simulink model "CryoDet12Chan"  (R2016b)
settings: Solver=ode45  StartTime=0.0  StopTime=10e-4  MaxStep=1e-9  RelTol=1e-3
values from neighbouring files (symbols this model uses):
  Fclk = Fadc/2    (= 153600000)    [setupCryoFPGA.m]    (also in setupCryoNew.m)
  freqBusAddrBits = 4    [setupCryoFPGA.m]    (also in setupCryoNew.m)
  noise = exp(2i*pi*rand(1, noiseLen))    [setupCryoFPGA.m]    (also in setupCryoNew.m)
  noiseLen = 128    [setupCryoFPGA.m]    (also in setupCryoNew.m)
  noiseSteps = 32    [setupCryoFPGA.m]    (also in setupCryoNew.m)
  notch = tf( [1 a*wNotch/Q wNotch^2], [1 wNotch/Q wNotch^2])    [setupCryoFPGA.m]    (also in setupCryoNew.m)
  notch2 = tf( [1 a*wNotch/Q wNotch^2], [1 wNotch/Q wNotch^2])    [setupCryoFPGA.m]    (also in setupCryoNew.m)
  notch3 = tf( [1 a*wNotch/Q wNotch^2], [1 wNotch/Q wNotch^2])    [setupCryoFPGA.m]    (also in setupCryoNew.m)
  notch4 = tf( [1 a*wNotch/Q wNotch^2], [1 wNotch/Q wNotch^2])    [setupCryoFPGA.m]    (also in setupCryoNew.m)
  Tclk = 1/Fclk    (= 6.51041666667e-09)    [setupCryoFPGA.m]    (also in setupCryoNew.m)
undefined symbols (not defined in the file or in its folder): AXI4, Lite, xlipgetpartsetting
libraries: xbsIndex_r4 x1191
(part 3 of 9)

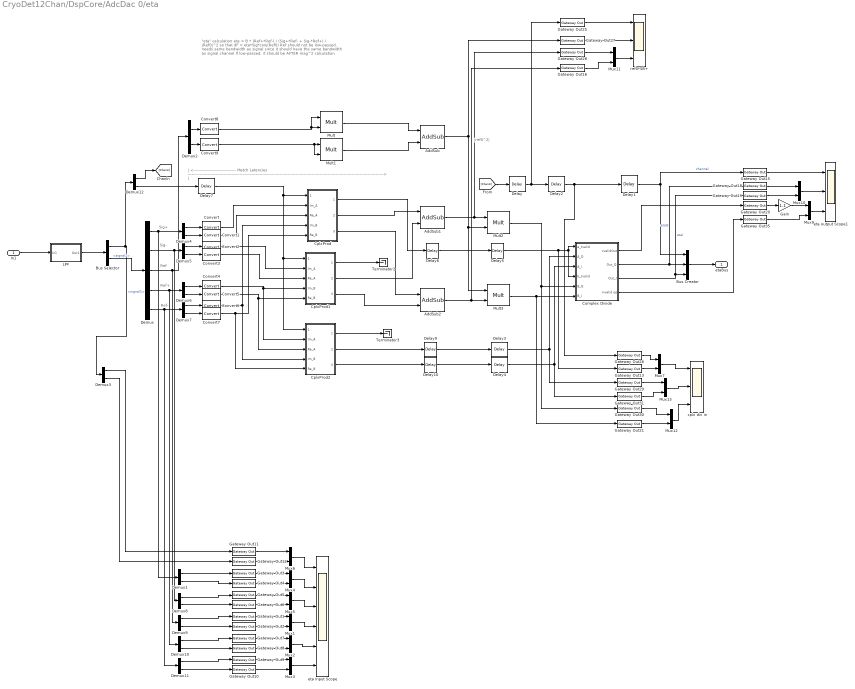
== system CryoDet12Chan/DspCore/AdcDac 0/eta ==
  note: Sig+
  note: Sig-
  note: Ref+
  note: "eta" calculation
      |
      | eta = B * (Ref+*Ref-) / (Sig+*Ref- + Sig-*Ref+) / |Ref0|^2
      |
      | so that dF = eta*Sig*conj(Ref0)
      |
      | Ref should not be low-passed, needs same bandwidth as signal since it should have the same bandwidth as signal channel
      | If low-passed, it should be AFTER mag^2 calculation
  note: Ref
  note: Ref-
  note: | <-------------------------------- Match Latencies ---------------------------------------------------------------------------------------------------------------------------------------------------> |
  note: |ref0^2|
  In1 : Inport
  AddSub : xbsIndex_r4/AddSub  mode=Addition  use_carryin=off  use_carryout=off  en=off  latency=3  precision=Full  arith_type=Unsigned  n_bits=32  bin_pt=30  quantization="Round  (unbiased: +/- Inf)"  overflow=Saturate  use_behavioral_HDL=off  hw_selection=DSP48  pipelined=on  dbl_ovrd=off  block_type=addsub
  AddSub1 : xbsIndex_r4/AddSub  mode=Addition  use_carryin=off  use_carryout=off  en=off  latency=3  precision=Full  arith_type="Signed  (2's comp)"  n_bits=32  bin_pt=30  quantization="Round  (unbiased: +/- Inf)"  overflow=Saturate  use_behavioral_HDL=off  hw_selection=DSP48  pipelined=on  dbl_ovrd=off  block_type=addsub
  AddSub2 : xbsIndex_r4/AddSub  mode=Addition  use_carryin=off  use_carryout=off  en=off  latency=3  precision=Full  arith_type="Signed  (2's comp)"  n_bits=32  bin_pt=30  quantization="Round  (unbiased: +/- Inf)"  overflow=Saturate  use_behavioral_HDL=off  hw_selection=DSP48  pipelined=on  dbl_ovrd=off  block_type=addsub
  Bus Creator : BusCreator  Inputs=3
  Bus Selector : BusSelector  OutputSignals=signal1,signal2
  Complex Divide : Subsystem
  Convert{,1..9} (10 alike) : xbsIndex_r4/Convert  gui_display_data_type=Floating-point  arith_type=Floating-point  n_bits=16  bin_pt=14  float_type=Single  exp_bits=8  fraction_bits=24  quantization=Truncate  overflow=Wrap  en=off  latency=1  pipeline=off  dbl_ovrd=off  block_type=convert
  CplxProd : Subsystem
  CplxProd1 : Subsystem
  CplxProd2 : Subsystem
  Delay : xbsIndex_r4/Delay  rst=off  infoeditControl=Selection of Reset will increase slice count due to use of real FFs and instead of SRLs  en=off  latency=10  reg_retiming=off  dbl_ovrd=off  block_type=delay
  Delay1 : xbsIndex_r4/Delay  rst=off  infoeditControl=Selection of Reset will increase slice count due to use of real FFs and instead of SRLs  en=off  latency=17  reg_retiming=on  dbl_ovrd=off  block_type=delay
  Delay{2..6,9..10} (7 alike) : xbsIndex_r4/Delay  rst=off  infoeditControl=Selection of Reset will increase slice count due to use of real FFs and instead of SRLs  en=off  latency=3  reg_retiming=off  dbl_ovrd=off  block_type=delay
  Delay7 : xbsIndex_r4/Delay  rst=off  infoeditControl=Selection of Reset will increase slice count due to use of real FFs and instead of SRLs  en=off  latency=1  reg_retiming=off  dbl_ovrd=off  block_type=delay
  Demux : Demux  Outputs=5
  Demux{1..12} (12 alike) : Demux  Outputs=2
  Gain : Gain  Gain=1.1
  Gateway Out{1..13,15..16,18..21,25..31,35} (27 alike) : xbsIndex_r4/Gateway Out  inherit_from_input=off  hdl_port=off  rows=1  columns=1  UseAsDAC=off  DACChannel='1'  interface=None  automatic_assignment=on  address_offset=hex2dec('00')  intf_name=''  intf_description=''  timing_constraint=None  locs_specified=off  LOCs={}  io_standard={}  block_type=gatewayout
  LPF : Subsystem
  Mult : xbsIndex_r4/Mult  precision=Full  arith_type="Signed  (2's comp)"  n_bits=32  bin_pt=30  quantization="Round  (unbiased: +/- Inf)"  overflow=Saturate  en=off  latency=6  use_behavioral_HDL=off  opt=Speed  use_embedded=on  optimum_pipeline=off  pipeline=on  dbl_ovrd=off  use_rpm=on  placement_style=Triangular  block_type=mult
  Mult1 : xbsIndex_r4/Mult  precision=Full  arith_type="Signed  (2's comp)"  n_bits=32  bin_pt=30  quantization="Round  (unbiased: +/- Inf)"  overflow=Saturate  en=off  latency=6  use_behavioral_HDL=off  opt=Speed  use_embedded=on  optimum_pipeline=off  pipeline=on  dbl_ovrd=off  use_rpm=on  placement_style=Triangular  block_type=mult
  Mult2 : xbsIndex_r4/Mult  precision=Full  arith_type="Signed  (2's comp)"  n_bits=32  bin_pt=30  quantization="Round  (unbiased: +/- Inf)"  overflow=Saturate  en=off  latency=3  use_behavioral_HDL=off  opt=Speed  use_embedded=on  optimum_pipeline=off  pipeline=on  dbl_ovrd=off  use_rpm=on  placement_style=Triangular  block_type=mult
  Mult3 : xbsIndex_r4/Mult  precision=Full  arith_type="Signed  (2's comp)"  n_bits=32  bin_pt=30  quantization="Round  (unbiased: +/- Inf)"  overflow=Saturate  en=off  latency=3  use_behavioral_HDL=off  opt=Speed  use_embedded=on  optimum_pipeline=off  pipeline=on  dbl_ovrd=off  use_rpm=on  placement_style=Triangular  block_type=mult
  Mux{1..7,9..13} (12 alike) : Mux  Inputs=2
  Terminator2 : Terminator
  Terminator3 : Terminator
  cplx div in : Scope  NumInputPorts=3
  eta Input Scope : Scope  NumInputPorts=6
  eta output Scope1 : Scope  NumInputPorts=3
  ref0*SB+ : Scope  NumInputPorts=3
  etaBus : Outport
  wires:
  Demux4/1 -> Convert/1
  Demux4/2 -> Convert1/1
  Demux7/1 -> Convert6/1
  Demux7/2 -> Convert7/1
  Demux5/1 -> Convert2/1
  Demux5/2 -> Convert3/1
  Demux6/1 -> Convert4/1
  Demux6/2 -> Convert5/1
  Demux12/2 -> Delay7/1
  AddSub2/1 -> Gateway Out16/1, Mult3/2
  AddSub1/1 -> Gateway Out28/1, Mult2/1
  Mult/1 -> AddSub/1
  Mult1/1 -> AddSub/2
  Demux2/1 -> Convert8/1
  Demux2/2 -> Convert9/1
  CplxProd1/3(Re_Out) -> AddSub2/2
  CplxProd/3(Re_Out) -> AddSub2/1
  CplxProd1/2(Im_Out) -> AddSub1/2
  AddSub/1 -> Mult3/1, Mult2/2, Gateway Out27/1
  Mult2/1 -> Complex Divide/5(B_Q), Gateway Out30/1
  Mult3/1 -> Gateway Out21/1, Complex Divide/6(B_I)
  CplxProd/1(tvalidOut) -> Delay6/1
  CplxProd2/3(Re_Out) -> Delay10/1
  In1/1 -> LPF/1(In1)
  Bus Selector/2 -> Demux/1  "<signal2>"
  [ChanIn] -> Delay/1
  Delay/1 -> Gateway Out25/1, Delay2/1
  LPF/1(Out1) -> Bus Selector/1
  Delay1/1 -> Gateway Out15/1, Bus Creator/1  "channel"
  Complex Divide/2(Out_Q) -> Gateway Out18/1, Bus Creator/2  "etaQ"
  Complex Divide/3(Out_I) -> Gateway Out19/1, Bus Creator/3  "etaI"
  Bus Creator/1 -> etaBus/1
  Bus Selector/1 -> Demux12/1, Demux3/1  "<signal1>"
  Demux3/1 -> Gateway Out11/1
  Demux3/2 -> Gateway Out12/1
  Demux/5 -> Demux11/1, Demux7/1
  Demux/4 -> Demux6/1, Demux10/1
  Demux/2 -> Demux8/1, Demux5/1
  Demux/1 -> Demux4/1, Demux1/1
  Demux/3 -> Demux9/1, Demux2/1
  CplxProd1/1(tvalidOut) -> Terminator2/1
  Gateway Out6/1 -> Mux5/2
  Gateway Out5/1 -> Mux5/1
  Gateway Out4/1 -> Mux4/2
  Gateway Out3/1 -> Mux4/1
  Mux4/1 -> eta Input Scope/2
  Mux5/1 -> eta Input Scope/3
  Gateway Out2/1 -> Mux1/2
  Gateway Out1/1 -> Mux1/1
  Gateway Out8/1 -> Mux2/2
  Gateway Out7/1 -> Mux2/1
  Gateway Out10/1 -> Mux3/2
  Gateway Out9/1 -> Mux3/1
  Mux3/1 -> eta Input Scope/6
  Mux2/1 -> eta Input Scope/5
  Mux1/1 -> eta Input Scope/4
  Demux1/1 -> Gateway Out3/1
  Demux1/2 -> Gateway Out4/1
  Demux8/2 -> Gateway Out6/1
  Demux8/1 -> Gateway Out5/1
  Demux9/2 -> Gateway Out2/1
  Demux9/1 -> Gateway Out1/1
  Demux10/2 -> Gateway Out8/1
  Demux10/1 -> Gateway Out7/1
  Demux11/2 -> Gateway Out10/1
  Demux11/1 -> Gateway Out9/1
  Gateway Out12/1 -> Mux6/2
  Gateway Out11/1 -> Mux6/1
  Mux6/1 -> eta Input Scope/1
  Gateway Out19/1 -> Mux10/2
  Gateway Out18/1 -> Mux10/1
  Mux10/1 -> eta output Scope1/2
  Gateway Out15/1 -> eta output Scope1/1
  Gateway Out25/1 -> ref0*SB+/1
  Gateway Out27/1 -> ref0*SB+/2
  Mux11/1 -> ref0*SB+/3
  Gateway Out28/1 -> Mux11/1
  Gateway Out16/1 -> Mux11/2
  Delay2/1 -> Gateway Out26/1, Delay1/1
  Delay3/1 -> Complex Divide/2(A_Q), Gateway Out29/1
  Delay4/1 -> Complex Divide/3(A_I), Gateway Out31/1
  Mux12/1 -> cplx div in/3
  Gateway Out30/1 -> Mux12/1
  Gateway Out21/1 -> Mux12/2
  Gateway Out29/1 -> Mux13/1
  Mux13/1 -> cplx div in/2
  Gateway Out31/1 -> Mux13/2
  Gateway Out13/1 -> Mux7/2
  Gateway Out26/1 -> Mux7/1
  Mux7/1 -> cplx div in/1
  Demux12/1 -> [ChanIn]
  CplxProd/2(Im_Out) -> AddSub1/1
  Gateway Out20/1 -> Gain/1
  Gateway Out35/1 -> Mux9/2
  Complex Divide/4(invalid op) -> Gateway Out35/1
  Mux9/1 -> eta output Scope1/3
  Gain/1 -> Mux9/1
  Convert/1 -> CplxProd/2(Im_A)
  Convert1/1 -> CplxProd/3(Re_A)
  Convert2/1 -> CplxProd1/2(Im_A)
  Convert3/1 -> CplxProd1/3(Re_A)
  Convert4/1 -> CplxProd2/2(Im_A), CplxProd1/4(Im_B)
  Convert5/1 -> CplxProd2/3(Re_A), CplxProd1/5(Re_B)
  Convert6/1 -> CplxProd2/4(Im_B), CplxProd/4(Im_B)
  Convert7/1 -> CplxProd2/5(Re_B), CplxProd/5(Re_B)
  Convert9/1 -> Mult1/2, Mult1/1
  Convert8/1 -> Mult/1, Mult/2
  Delay6/1 -> Delay5/1
  Delay7/1 -> CplxProd/1(tvalidIn), CplxProd1/1(tvalidIn), CplxProd2/1(tvalidIn)
  CplxProd2/1(tvalidOut) -> Terminator3/1
  Delay10/1 -> Delay4/1
  Delay9/1 -> Delay3/1
  CplxProd2/2(Im_Out) -> Delay9/1
  Delay5/1 -> Gateway Out13/1, Complex Divide/4(b_tvalid), Complex Divide/1(a_tvalid)
  Complex Divide/1(tvalidOut) -> Gateway Out20/1

== system CryoDet12Chan/DspCore/AdcDac 0/loopFilter ==
  note: convert to MHz
  note: F out should be Fi + DF
      | where DF is integral of frequency error dF subject to limits and FBen
  note: loopFilter
      | multi-line feedback block
      | mplement intial frequency, limits, integrator, gain
  In1 : Inport
  Assert : xbsIndex_r4/Assert  assert_type=on  type_source=Explicitly  gui_display_data_type=Fixed-point  arith_type=Unsigned  n_bits=4  bin_pt=0  preci_type=Single  exp_width=8  frac_width=24  assert_rate=on  rate_source=Explicitly  period=Tclk  output_port=on  block_type=assert
  Assert1 : xbsIndex_r4/Assert  assert_type=on  type_source=Explicitly  gui_display_data_type=Fixed-point  arith_type="Signed  (2's comp)"  n_bits=32  bin_pt=30  preci_type=Single  exp_width=8  frac_width=24  assert_rate=on  rate_source=Explicitly  period=Tclk  output_port=on  block_type=assert
  Assert2 : xbsIndex_r4/Assert  assert_type=on  type_source=Explicitly  gui_display_data_type=Boolean  arith_type=Boolean  n_bits=16  bin_pt=14  preci_type=Single  exp_width=8  frac_width=24  assert_rate=on  rate_source=Explicitly  period=Tclk  output_port=on  block_type=assert
  Assert5 : xbsIndex_r4/Assert  assert_type=on  type_source=Explicitly  gui_display_data_type=Fixed-point  arith_type=Unsigned  n_bits=25  bin_pt=0  preci_type=Single  exp_width=8  frac_width=24  assert_rate=on  rate_source=Explicitly  period=Tclk  output_port=on  block_type=assert
  Assert6 : xbsIndex_r4/Assert  assert_type=on  type_source=Explicitly  gui_display_data_type=Fixed-point  arith_type=Unsigned  n_bits=16  bin_pt=16  preci_type=Single  exp_width=8  frac_width=24  assert_rate=on  rate_source=Explicitly  period=Tclk  output_port=on  block_type=assert
  Assert8 : xbsIndex_r4/Assert  assert_type=on  type_source=Explicitly  gui_display_data_type=Fixed-point  arith_type=Unsigned  n_bits=24  bin_pt=24  preci_type=Single  exp_width=8  frac_width=24  assert_rate=on  rate_source=Explicitly  period=Tclk  output_port=on  block_type=assert
  Assert9 : xbsIndex_r4/Assert  assert_type=on  type_source=Explicitly  gui_display_data_type=Fixed-point  arith_type=Unsigned  n_bits=4  bin_pt=0  preci_type=Single  exp_width=8  frac_width=24  assert_rate=on  rate_source=Explicitly  period=Tclk  output_port=on  block_type=assert
  Bus Selector : BusSelector  OutputSignals=channel,freqError
  Concat : xbsIndex_r4/Concat  num_inputs=2  dbl_ovrd=off  block_type=concat
  Constant : xbsIndex_r4/Constant  const=0  gui_display_data_type=Fixed-point  arith_type=Unsigned  n_bits=4  bin_pt=0  preci_type=Single  exp_width=8  frac_width=24  explicit_period=off  period=1  equ=P=C  opselect=C  inp2=PCIN>>17  opr=+  inp1=P  carry=CIN  dbl_ovrd=off  block_type=constant
  Constant1 : xbsIndex_r4/Constant  const=0  gui_display_data_type=Fixed-point  arith_type=Unsigned  n_bits=4  bin_pt=0  preci_type=Single  exp_width=8  frac_width=24  explicit_period=off  period=1  equ=P=C  opselect=C  inp2=PCIN>>17  opr=+  inp1=P  carry=CIN  dbl_ovrd=off  block_type=constant
  Constant2 : xbsIndex_r4/Constant  const=1  gui_display_data_type=Fixed-point  arith_type=Unsigned  n_bits=4  bin_pt=0  preci_type=Single  exp_width=8  frac_width=24  explicit_period=off  period=1  equ=P=C  opselect=C  inp2=PCIN>>17  opr=+  inp1=P  carry=CIN  dbl_ovrd=off  block_type=constant
  Delay2 : xbsIndex_r4/Delay  rst=off  infoeditControl=Selection of Reset will increase slice count due to use of real FFs and instead of SRLs  en=off  latency=3  reg_retiming=off  dbl_ovrd=off  block_type=delay
  Delay3 : xbsIndex_r4/Delay  rst=off  infoeditControl=Selection of Reset will increase slice count due to use of real FFs and instead of SRLs  en=off  latency=3  reg_retiming=off  dbl_ovrd=off  block_type=delay
  Display2 : Display
  Display3 : Display
  Gain1 : Gain  Gain=185
  Gain2 : Gain  Gain=185
  Gain3 : Gain  Gain=185
  Gateway Out12 : xbsIndex_r4/Gateway Out  inherit_from_input=off  hdl_port=off  rows=1  columns=1  UseAsDAC=off  DACChannel='1'  interface=None  automatic_assignment=on  address_offset=hex2dec('00')  intf_name=''  intf_description=''  timing_constraint=None  locs_specified=off  LOCs={}  io_standard={}  block_type=gatewayout
  Gateway Out13 : xbsIndex_r4/Gateway Out  inherit_from_input=on  hdl_port=off  rows=1  columns=1  UseAsDAC=off  DACChannel='1'  interface=None  automatic_assignment=on  address_offset=hex2dec('00')  intf_name=''  intf_description=''  timing_constraint=None  locs_specified=off  LOCs={}  io_standard={}  block_type=gatewayout
  Gateway Out3 : xbsIndex_r4/Gateway Out  inherit_from_input=off  hdl_port=off  rows=1  columns=1  UseAsDAC=off  DACChannel='1'  interface=None  automatic_assignment=on  address_offset=hex2dec('00')  intf_name=''  intf_description=''  timing_constraint=None  locs_specified=off  LOCs={}  io_standard={}  block_type=gatewayout
  Gateway Out4 : xbsIndex_r4/Gateway Out  inherit_from_input=off  hdl_port=off  rows=1  columns=1  UseAsDAC=off  DACChannel='1'  interface=None  automatic_assignment=on  address_offset=hex2dec('00')  intf_name=''  intf_description=''  timing_constraint=None  locs_specified=off  LOCs={}  io_standard={}  block_type=gatewayout
  Gateway Out5 : xbsIndex_r4/Gateway Out  inherit_from_input=on  hdl_port=off  rows=1  columns=1  UseAsDAC=off  DACChannel='1'  interface=None  automatic_assignment=on  address_offset=hex2dec('00')  intf_name=''  intf_description=''  timing_constraint=None  locs_specified=off  LOCs={}  io_standard={}  block_type=gatewayout
  Logical : xbsIndex_r4/Logical  logical_function=OR  inputs=2  en=off  latency=3  precision=User Defined  arith_type=Boolean  n_bits=16  bin_pt=0  align_bp=on  dbl_ovrd=off  block_type=logical
  MCode : xbsIndex_r4/MCode  mfname=multiLineFeedbackpipelined  explicit_period=on  period=Tclk  inputsTable={'boundInpExpr'=>['','','','',''],'inputs'=>['channelNo','deltaF','FBen','Finitial','dFmax']}  outputsTable={'outputs'=>['freq','chanOut'],'suppressOut'=>['off','off']}  enable_stdout=off  enable_debug=off  suppress_output=on  defparams={}  hide_port_list={}  dbl_ovrd=off  block_type=mcode
  Mult : xbsIndex_r4/Mult  precision=User Defined  arith_type="Signed  (2's comp)"  n_bits=32  bin_pt=30  quantization=Truncate  overflow=Saturate  en=off  latency=3  use_behavioral_HDL=off  opt=Speed  use_embedded=on  optimum_pipeline=off  pipeline=on  dbl_ovrd=off  use_rpm=on  placement_style=Triangular  block_type=mult
  Mux : xbsIndex_r4/Mux  inputs=2  en=off  latency=1  precision=Full  arith_type=Unsigned  n_bits=16  bin_pt=14  quantization=Truncate  overflow=Wrap  dbl_ovrd=off  block_type=mux
  Negate : xbsIndex_r4/Negate  precision=Full  arith_type=Unsigned  n_bits=16  bin_pt=14  quantization=Truncate  overflow=Wrap  en=off  latency=1  dbl_ovrd=off  block_type=negate
  Register : xbsIndex_r4/Register  init=0  rst=off  en=on  dbl_ovrd=off  block_type=register
  Register1 : xbsIndex_r4/Register  init=0  rst=off  en=on  dbl_ovrd=off  block_type=register
  Register2 : xbsIndex_r4/Register  init=0  rst=off  en=on  dbl_ovrd=off  block_type=register
  Reinterpret : xbsIndex_r4/Reinterpret  force_arith_type=off  arith_type=Unsigned  force_bin_pt=on  bin_pt=0  block_type=reinterpret
  Relational : xbsIndex_r4/Relational  mode=a=b  op_type=Bool  en=off  latency=0  dbl_ovrd=off  block_type=relational
  Relational1 : xbsIndex_r4/Relational  mode=a=b  op_type=Bool  en=off  latency=0  dbl_ovrd=off  block_type=relational
  Relational2 : xbsIndex_r4/Relational  mode=a=b  op_type=Bool  en=off  latency=0  dbl_ovrd=off  block_type=relational
  initial Frequencies : Subsystem
  loop filter input : Scope  NumInputPorts=2
  loop filter output : Scope  NumInputPorts=3
  Out1 : Outport
  tag scope: freqBus=global
  wires:
  In1/1 -> Bus Selector/1
  Bus Selector/1 -> Relational/1, Gateway Out3/1, initial Frequencies/1(channel), Delay3/1  "<channel>"
  Bus Selector/2 -> Mult/1, Register/1  "<freqError>"
  MCode/2 -> Assert9/1, Relational2/2, Gateway Out12/1, Relational1/2  "channel"
  MCode/1 -> Assert8/1, Register2/1, Register1/1  "frequency"
  Concat/1 -> [freqBus], Out1/1
  [fbPolarity] -> Mux/1
  [FBgain] -> Mux/2, Negate/1
  [FBlimit] -> Assert6/1
  initial Frequencies/1(Fi) -> Delay2/1
  Assert/1 -> MCode/1
  Assert1/1 -> MCode/2
  Assert2/1 -> MCode/3
  Assert5/1 -> MCode/4
  Assert6/1 -> MCode/5
  Assert9/1 -> Concat/1
  Assert8/1 -> Reinterpret/1
  Reinterpret/1 -> Concat/2
  Gateway Out13/1 -> Gain1/1
  Gateway Out12/1 -> loop filter output/1
  Gateway Out4/1 -> Gain2/1
  Gateway Out3/1 -> loop filter input/1, Display2/1
  Constant/1 -> Relational/2
  Relational/1 -> Register/2
  Register/1 -> Gateway Out4/1
  Constant1/1 -> Relational1/1
  Relational1/1 -> Register1/2
  Register1/1 -> Gateway Out13/1
  Gain1/1 -> loop filter output/2
  Gain2/1 -> Display3/1, loop filter input/2
  Constant2/1 -> Relational2/1
  Relational2/1 -> Register2/2
  Register2/1 -> Gateway Out5/1
  Gateway Out5/1 -> Gain3/1
  Gain3/1 -> loop filter output/3
  Negate/1 -> Mux/3
  Mult/1 -> Assert1/1
  Mux/1 -> Mult/2
  [fpgaReset] -> Logical/2
  [FBen] -> Logical/1
  Logical/1 -> Assert2/1
  Delay3/1 -> Assert/1
  Delay2/1 -> Assert5/1

== system CryoDet12Chan/DspCore/AdcDac 0/twelveLineUDC 0 ==
  In1 : Inport
  BDC scope : Scope  NumInputPorts=2
  Constant : xbsIndex_r4/Constant  const=0  gui_display_data_type=Fixed-point  arith_type=Unsigned  n_bits=4  bin_pt=0  preci_type=Single  exp_width=8  frac_width=24  explicit_period=off  period=1  equ=P=C  opselect=C  inp2=PCIN>>17  opr=+  inp1=P  carry=CIN  dbl_ovrd=off  block_type=constant
  Constant1 : xbsIndex_r4/Constant  const=1  gui_display_data_type=Fixed-point  arith_type=Unsigned  n_bits=4  bin_pt=0  preci_type=Single  exp_width=8  frac_width=24  explicit_period=off  period=1  equ=P=C  opselect=C  inp2=PCIN>>17  opr=+  inp1=P  carry=CIN  dbl_ovrd=off  block_type=constant
  Constant10 : xbsIndex_r4/Constant  const=10  gui_display_data_type=Fixed-point  arith_type=Unsigned  n_bits=4  bin_pt=0  preci_type=Single  exp_width=8  frac_width=24  explicit_period=off  period=1  equ=P=C  opselect=C  inp2=PCIN>>17  opr=+  inp1=P  carry=CIN  dbl_ovrd=off  block_type=constant
  Constant11 : xbsIndex_r4/Constant  const=11  gui_display_data_type=Fixed-point  arith_type=Unsigned  n_bits=4  bin_pt=0  preci_type=Single  exp_width=8  frac_width=24  explicit_period=off  period=1  equ=P=C  opselect=C  inp2=PCIN>>17  opr=+  inp1=P  carry=CIN  dbl_ovrd=off  block_type=constant
  Constant12 : xbsIndex_r4/Constant  const=15  gui_display_data_type=Fixed-point  arith_type=Unsigned  n_bits=4  bin_pt=0  preci_type=Single  exp_width=8  frac_width=24  explicit_period=off  period=1  equ=P=C  opselect=C  inp2=PCIN>>17  opr=+  inp1=P  carry=CIN  dbl_ovrd=off  block_type=constant
  Constant2 : xbsIndex_r4/Constant  const=2  gui_display_data_type=Fixed-point  arith_type=Unsigned  n_bits=4  bin_pt=0  preci_type=Single  exp_width=8  frac_width=24  explicit_period=off  period=1  equ=P=C  opselect=C  inp2=PCIN>>17  opr=+  inp1=P  carry=CIN  dbl_ovrd=off  block_type=constant
  Constant3 : xbsIndex_r4/Constant  const=3  gui_display_data_type=Fixed-point  arith_type=Unsigned  n_bits=4  bin_pt=0  preci_type=Single  exp_width=8  frac_width=24  explicit_period=off  period=1  equ=P=C  opselect=C  inp2=PCIN>>17  opr=+  inp1=P  carry=CIN  dbl_ovrd=off  block_type=constant
  Constant4 : xbsIndex_r4/Constant  const=4  gui_display_data_type=Fixed-point  arith_type=Unsigned  n_bits=4  bin_pt=0  preci_type=Single  exp_width=8  frac_width=24  explicit_period=off  period=1  equ=P=C  opselect=C  inp2=PCIN>>17  opr=+  inp1=P  carry=CIN  dbl_ovrd=off  block_type=constant
  Constant5 : xbsIndex_r4/Constant  const=5  gui_display_data_type=Fixed-point  arith_type=Unsigned  n_bits=4  bin_pt=0  preci_type=Single  exp_width=8  frac_width=24  explicit_period=off  period=1  equ=P=C  opselect=C  inp2=PCIN>>17  opr=+  inp1=P  carry=CIN  dbl_ovrd=off  block_type=constant
  Constant6 : xbsIndex_r4/Constant  const=6  gui_display_data_type=Fixed-point  arith_type=Unsigned  n_bits=4  bin_pt=0  preci_type=Single  exp_width=8  frac_width=24  explicit_period=off  period=1  equ=P=C  opselect=C  inp2=PCIN>>17  opr=+  inp1=P  carry=CIN  dbl_ovrd=off  block_type=constant
  Constant7 : xbsIndex_r4/Constant  const=7  gui_display_data_type=Fixed-point  arith_type=Unsigned  n_bits=4  bin_pt=0  preci_type=Single  exp_width=8  frac_width=24  explicit_period=off  period=1  equ=P=C  opselect=C  inp2=PCIN>>17  opr=+  inp1=P  carry=CIN  dbl_ovrd=off  block_type=constant
  Constant8 : xbsIndex_r4/Constant  const=8  gui_display_data_type=Fixed-point  arith_type=Unsigned  n_bits=4  bin_pt=0  preci_type=Single  exp_width=8  frac_width=24  explicit_period=off  period=1  equ=P=C  opselect=C  inp2=PCIN>>17  opr=+  inp1=P  carry=CIN  dbl_ovrd=off  block_type=constant
  Constant9 : xbsIndex_r4/Constant  const=9  gui_display_data_type=Fixed-point  arith_type=Unsigned  n_bits=4  bin_pt=0  preci_type=Single  exp_width=8  frac_width=24  explicit_period=off  period=1  equ=P=C  opselect=C  inp2=PCIN>>17  opr=+  inp1=P  carry=CIN  dbl_ovrd=off  block_type=constant
  Counter : xbsIndex_r4/Counter  cnt_type=Count Limited  cnt_to=15  operation=Up  start_count=0  cnt_by_val=1  arith_type=Unsigned  n_bits=4  bin_pt=0  load_pin=off  rst=on  en=on  explicit_period=off  period=Tclk  use_behavioral_HDL=off  implementation=Fabric  dbl_ovrd=off  block_type=counter
  DAC Sum : Subsystem
  Delay : xbsIndex_r4/Delay  rst=off  infoeditControl=Selection of Reset will increase slice count due to use of real FFs and instead of SRLs  en=off  latency=6  reg_retiming=off  dbl_ovrd=off  block_type=delay
  Demux : Demux
  Gateway Out{1,7..10,23} (6 alike) : xbsIndex_r4/Gateway Out  inherit_from_input=off  hdl_port=off  rows=1  columns=1  UseAsDAC=off  DACChannel='1'  interface=None  automatic_assignment=on  address_offset=hex2dec('00')  intf_name=''  intf_description=''  timing_constraint=None  locs_specified=off  LOCs={}  io_standard={}  block_type=gatewayout
  Mux12X4 : Subsystem
  Mux6 : Mux  Inputs=2
  Mux7 : Mux  Inputs=2
  Relational : xbsIndex_r4/Relational  mode=a!=b  op_type=Bool  en=off  latency=0  dbl_ovrd=off  block_type=relational
  SBdemod : Subsystem
  Toolbar : xbsIndex_r4/Toolbar  func=xltoolbar  block_type=toolbar
      settings: infoedit=Toolbar
  oneLineUpDown0 : Subsystem
  oneLineUpDown1 : Subsystem
  oneLineUpDown10 : Subsystem
  oneLineUpDown11 : Subsystem
  oneLineUpDown2 : Subsystem
  oneLineUpDown3 : Subsystem
  oneLineUpDown4 : Subsystem
  oneLineUpDown5 : Subsystem
  oneLineUpDown6 : Subsystem
  oneLineUpDown7 : Subsystem
  oneLineUpDown8 : Subsystem
  oneLineUpDown9 : Subsystem
  synch scope : Scope  NumInputPorts=2
  toDAC : Outport
  demodulated : Outport  Port=2
  wires:
  [fpgaReset] -> Counter/1, Delay/1
  oneLineUpDown7/1(Out1) -> Mux12X4/8(line7)
  oneLineUpDown6/1(Out1) -> Mux12X4/7(line6)
  oneLineUpDown5/1(Out1) -> Mux12X4/6(line5)
  oneLineUpDown4/1(Out1) -> Mux12X4/5(line4)
  oneLineUpDown3/1(Out1) -> Mux12X4/4(line3)
  oneLineUpDown2/1(Out1) -> Mux12X4/3(line2)
  Mux12X4/1(Out1) -> SBdemod/1(In1)
  oneLineUpDown1/1(Out1) -> Mux12X4/2(line1)
  oneLineUpDown0/1(Out1) -> Mux12X4/1(line0)
  oneLineUpDown8/1(Out1) -> Mux12X4/9(line8)
  oneLineUpDown9/1(Out1) -> Mux12X4/10(line9)
  oneLineUpDown10/1(Out1) -> Mux12X4/11(line10)
  oneLineUpDown11/1(Out1) -> Mux12X4/12(line11)
  oneLineUpDown11/2(toDAC) -> DAC Sum/12(In12)
  oneLineUpDown10/2(toDAC) -> DAC Sum/11(In11)
  oneLineUpDown9/2(toDAC) -> DAC Sum/10(In10)
  oneLineUpDown8/2(toDAC) -> DAC Sum/9(In9)
  oneLineUpDown7/2(toDAC) -> DAC Sum/8(In8)
  oneLineUpDown6/2(toDAC) -> DAC Sum/7(In7)
  oneLineUpDown5/2(toDAC) -> DAC Sum/6(In6)
  oneLineUpDown4/2(toDAC) -> DAC Sum/5(In5)
  oneLineUpDown3/2(toDAC) -> DAC Sum/4(In4)
  oneLineUpDown2/2(toDAC) -> DAC Sum/3(In3)
  oneLineUpDown1/2(toDAC) -> DAC Sum/2(In2)
  oneLineUpDown0/2(toDAC) -> DAC Sum/1(In1)
  DAC Sum/1(Out1) -> toDAC/1
  SBdemod/1(AllComponents) -> demodulated/1
  Gateway Out10/1 -> Mux7/2
  Gateway Out9/1 -> Mux7/1
  Gateway Out8/1 -> Mux6/2
  Gateway Out7/1 -> Mux6/1
  Mux6/1 -> BDC scope/1
  Mux7/1 -> BDC scope/2
  Demux/1 -> Gateway Out7/1
  Demux/4 -> Gateway Out10/1
  Demux/3 -> Gateway Out9/1
  Demux/2 -> Gateway Out8/1
  Delay/1 -> Mux12X4/13(synch)
  Constant/1 -> oneLineUpDown0/2(addrIn)
  Constant1/1 -> oneLineUpDown1/2(addrIn)
  Constant2/1 -> oneLineUpDown2/2(addrIn)
  Constant3/1 -> oneLineUpDown3/2(addrIn)
  Constant4/1 -> oneLineUpDown4/2(addrIn)
  Constant5/1 -> oneLineUpDown5/2(addrIn)
  Constant6/1 -> oneLineUpDown6/2(addrIn)
  Constant7/1 -> oneLineUpDown7/2(addrIn)
  Constant8/1 -> oneLineUpDown8/2(addrIn)
  Constant9/1 -> oneLineUpDown9/2(addrIn)
  Constant10/1 -> oneLineUpDown10/2(addrIn)
  Constant11/1 -> oneLineUpDown11/2(addrIn)
  In1/1 -> oneLineUpDown6/1(In), oneLineUpDown8/1(In), oneLineUpDown9/1(In), oneLineUpDown10/1(In), oneLineUpDown11/1(In), oneLineUpDown7/1(In), Demux/1, oneLineUpDown5/1(In), oneLineUpDown4/1(In), oneLineUpDown3/1(In), oneLineUpDown2/1(In), oneLineUpDown1/1(In), oneLineUpDown0/1(In)
  Counter/1 -> Gateway Out23/1, Relational/2, oneLineUpDown2/3(synchIn), oneLineUpDown3/3(synchIn), oneLineUpDown4/3(synchIn), oneLineUpDown5/3(synchIn), oneLineUpDown6/3(synchIn), oneLineUpDown7/3(synchIn), oneLineUpDown8/3(synchIn), oneLineUpDown10/3(synchIn), oneLineUpDown11/3(synchIn), oneLineUpDown9/3(synchIn), oneLineUpDown1/3(synchIn), oneLineUpDown0/3(synchIn)
  Gateway Out23/1 -> synch scope/1
  Gateway Out1/1 -> synch scope/2
  Relational/1 -> Gateway Out1/1, Counter/2
  Constant12/1 -> Relational/1

== system CryoDet12Chan/DspCore/AdcDac 0/twelveLineUDC 1 ==
  note: Null for now, eventually copy twelveLineUDC 0
      | when we need more than 12 lines per ADC channel
  In1 : Inport
  Out1 : Outport
  wires:
  In1/1 -> Out1/1

== system CryoDet12Chan/DspCore/Status & Debug/Addr Decode ==
  In1 : Inport
  Constant : xbsIndex_r4/Constant  const=0  gui_display_data_type=Fixed-point  arith_type=Unsigned  n_bits=4  bin_pt=0  preci_type=Single  exp_width=8  frac_width=24  explicit_period=off  period=1  equ=P=C  opselect=C  inp2=PCIN>>17  opr=+  inp1=P  carry=CIN  dbl_ovrd=off  block_type=constant
  Constant1 : xbsIndex_r4/Constant  const=1  gui_display_data_type=Fixed-point  arith_type=Unsigned  n_bits=4  bin_pt=0  preci_type=Single  exp_width=8  frac_width=24  explicit_period=off  period=1  equ=P=C  opselect=C  inp2=PCIN>>17  opr=+  inp1=P  carry=CIN  dbl_ovrd=off  block_type=constant
  Constant10 : xbsIndex_r4/Constant  const=10  gui_display_data_type=Fixed-point  arith_type=Unsigned  n_bits=4  bin_pt=0  preci_type=Single  exp_width=8  frac_width=24  explicit_period=off  period=1  equ=P=C  opselect=C  inp2=PCIN>>17  opr=+  inp1=P  carry=CIN  dbl_ovrd=off  block_type=constant
  Constant11 : xbsIndex_r4/Constant  const=11  gui_display_data_type=Fixed-point  arith_type=Unsigned  n_bits=4  bin_pt=0  preci_type=Single  exp_width=8  frac_width=24  explicit_period=off  period=1  equ=P=C  opselect=C  inp2=PCIN>>17  opr=+  inp1=P  carry=CIN  dbl_ovrd=off  block_type=constant
  Constant2 : xbsIndex_r4/Constant  const=2  gui_display_data_type=Fixed-point  arith_type=Unsigned  n_bits=4  bin_pt=0  preci_type=Single  exp_width=8  frac_width=24  explicit_period=off  period=1  equ=P=C  opselect=C  inp2=PCIN>>17  opr=+  inp1=P  carry=CIN  dbl_ovrd=off  block_type=constant
  Constant3 : xbsIndex_r4/Constant  const=3  gui_display_data_type=Fixed-point  arith_type=Unsigned  n_bits=4  bin_pt=0  preci_type=Single  exp_width=8  frac_width=24  explicit_period=off  period=1  equ=P=C  opselect=C  inp2=PCIN>>17  opr=+  inp1=P  carry=CIN  dbl_ovrd=off  block_type=constant
  Constant4 : xbsIndex_r4/Constant  const=4  gui_display_data_type=Fixed-point  arith_type=Unsigned  n_bits=4  bin_pt=0  preci_type=Single  exp_width=8  frac_width=24  explicit_period=off  period=1  equ=P=C  opselect=C  inp2=PCIN>>17  opr=+  inp1=P  carry=CIN  dbl_ovrd=off  block_type=constant
  Constant5 : xbsIndex_r4/Constant  const=5  gui_display_data_type=Fixed-point  arith_type=Unsigned  n_bits=4  bin_pt=0  preci_type=Single  exp_width=8  frac_width=24  explicit_period=off  period=1  equ=P=C  opselect=C  inp2=PCIN>>17  opr=+  inp1=P  carry=CIN  dbl_ovrd=off  block_type=constant
  Constant6 : xbsIndex_r4/Constant  const=6  gui_display_data_type=Fixed-point  arith_type=Unsigned  n_bits=4  bin_pt=0  preci_type=Single  exp_width=8  frac_width=24  explicit_period=off  period=1  equ=P=C  opselect=C  inp2=PCIN>>17  opr=+  inp1=P  carry=CIN  dbl_ovrd=off  block_type=constant
  Constant7 : xbsIndex_r4/Constant  const=7  gui_display_data_type=Fixed-point  arith_type=Unsigned  n_bits=4  bin_pt=0  preci_type=Single  exp_width=8  frac_width=24  explicit_period=off  period=1  equ=P=C  opselect=C  inp2=PCIN>>17  opr=+  inp1=P  carry=CIN  dbl_ovrd=off  block_type=constant
  Constant8 : xbsIndex_r4/Constant  const=8  gui_display_data_type=Fixed-point  arith_type=Unsigned  n_bits=4  bin_pt=0  preci_type=Single  exp_width=8  frac_width=24  explicit_period=off  period=1  equ=P=C  opselect=C  inp2=PCIN>>17  opr=+  inp1=P  carry=CIN  dbl_ovrd=off  block_type=constant
  Constant9 : xbsIndex_r4/Constant  const=9  gui_display_data_type=Fixed-point  arith_type=Unsigned  n_bits=4  bin_pt=0  preci_type=Single  exp_width=8  frac_width=24  explicit_period=off  period=1  equ=P=C  opselect=C  inp2=PCIN>>17  opr=+  inp1=P  carry=CIN  dbl_ovrd=off  block_type=constant
  Relational{2..13} (12 alike) : xbsIndex_r4/Relational  mode=a=b  op_type=Bool  en=off  latency=0  dbl_ovrd=off  block_type=relational
  Out1 : Outport
  Out2 : Outport  Port=2
  Out3 : Outport  Port=3
  Out4 : Outport  Port=4
  Out5 : Outport  Port=5
  Out6 : Outport  Port=6
  Out7 : Outport  Port=7
  Out8 : Outport  Port=8
  Out9 : Outport  Port=9
  Out10 : Outport  Port=10
  Out11 : Outport  Port=11
  Out12 : Outport  Port=12
  wires:
  Constant1/1 -> Relational3/2
  Constant2/1 -> Relational4/2
  Relational2/1 -> Out1/1
  Relational5/1 -> Out4/1
  Relational6/1 -> Out5/1
  Relational12/1 -> Out11/1
  Relational7/1 -> Out6/1
  Relational11/1 -> Out10/1
  Relational10/1 -> Out9/1
  Relational13/1 -> Out12/1
  Constant/1 -> Relational2/2
  Constant4/1 -> Relational6/2
  Constant5/1 -> Relational7/2
  Constant6/1 -> Relational8/2
  Constant7/1 -> Relational9/2
  Constant3/1 -> Relational5/2
  Constant9/1 -> Relational11/2
  Constant8/1 -> Relational10/2
  Constant10/1 -> Relational12/2
  Constant11/1 -> Relational13/2
  Relational8/1 -> Out7/1
  Relational4/1 -> Out3/1
  Relational3/1 -> Out2/1
  Relational9/1 -> Out8/1
  In1/1 -> Relational3/1, Relational4/1, Relational6/1, Relational7/1, Relational8/1, Relational9/1, Relational10/1, Relational11/1, Relational12/1, Relational13/1, Relational5/1, Relational2/1

== system CryoDet12Chan/DspCore/Status & Debug/Addr Decode1 ==
  In1 : Inport
  Constant : xbsIndex_r4/Constant  const=0  gui_display_data_type=Fixed-point  arith_type=Unsigned  n_bits=4  bin_pt=0  preci_type=Single  exp_width=8  frac_width=24  explicit_period=off  period=1  equ=P=C  opselect=C  inp2=PCIN>>17  opr=+  inp1=P  carry=CIN  dbl_ovrd=off  block_type=constant
  Constant1 : xbsIndex_r4/Constant  const=1  gui_display_data_type=Fixed-point  arith_type=Unsigned  n_bits=4  bin_pt=0  preci_type=Single  exp_width=8  frac_width=24  explicit_period=off  period=1  equ=P=C  opselect=C  inp2=PCIN>>17  opr=+  inp1=P  carry=CIN  dbl_ovrd=off  block_type=constant
  Constant10 : xbsIndex_r4/Constant  const=10  gui_display_data_type=Fixed-point  arith_type=Unsigned  n_bits=4  bin_pt=0  preci_type=Single  exp_width=8  frac_width=24  explicit_period=off  period=1  equ=P=C  opselect=C  inp2=PCIN>>17  opr=+  inp1=P  carry=CIN  dbl_ovrd=off  block_type=constant
  Constant11 : xbsIndex_r4/Constant  const=11  gui_display_data_type=Fixed-point  arith_type=Unsigned  n_bits=4  bin_pt=0  preci_type=Single  exp_width=8  frac_width=24  explicit_period=off  period=1  equ=P=C  opselect=C  inp2=PCIN>>17  opr=+  inp1=P  carry=CIN  dbl_ovrd=off  block_type=constant
  Constant2 : xbsIndex_r4/Constant  const=2  gui_display_data_type=Fixed-point  arith_type=Unsigned  n_bits=4  bin_pt=0  preci_type=Single  exp_width=8  frac_width=24  explicit_period=off  period=1  equ=P=C  opselect=C  inp2=PCIN>>17  opr=+  inp1=P  carry=CIN  dbl_ovrd=off  block_type=constant
  Constant3 : xbsIndex_r4/Constant  const=3  gui_display_data_type=Fixed-point  arith_type=Unsigned  n_bits=4  bin_pt=0  preci_type=Single  exp_width=8  frac_width=24  explicit_period=off  period=1  equ=P=C  opselect=C  inp2=PCIN>>17  opr=+  inp1=P  carry=CIN  dbl_ovrd=off  block_type=constant
  Constant4 : xbsIndex_r4/Constant  const=4  gui_display_data_type=Fixed-point  arith_type=Unsigned  n_bits=4  bin_pt=0  preci_type=Single  exp_width=8  frac_width=24  explicit_period=off  period=1  equ=P=C  opselect=C  inp2=PCIN>>17  opr=+  inp1=P  carry=CIN  dbl_ovrd=off  block_type=constant
  Constant5 : xbsIndex_r4/Constant  const=5  gui_display_data_type=Fixed-point  arith_type=Unsigned  n_bits=4  bin_pt=0  preci_type=Single  exp_width=8  frac_width=24  explicit_period=off  period=1  equ=P=C  opselect=C  inp2=PCIN>>17  opr=+  inp1=P  carry=CIN  dbl_ovrd=off  block_type=constant
  Constant6 : xbsIndex_r4/Constant  const=6  gui_display_data_type=Fixed-point  arith_type=Unsigned  n_bits=4  bin_pt=0  preci_type=Single  exp_width=8  frac_width=24  explicit_period=off  period=1  equ=P=C  opselect=C  inp2=PCIN>>17  opr=+  inp1=P  carry=CIN  dbl_ovrd=off  block_type=constant
  Constant7 : xbsIndex_r4/Constant  const=7  gui_display_data_type=Fixed-point  arith_type=Unsigned  n_bits=4  bin_pt=0  preci_type=Single  exp_width=8  frac_width=24  explicit_period=off  period=1  equ=P=C  opselect=C  inp2=PCIN>>17  opr=+  inp1=P  carry=CIN  dbl_ovrd=off  block_type=constant
  Constant8 : xbsIndex_r4/Constant  const=8  gui_display_data_type=Fixed-point  arith_type=Unsigned  n_bits=4  bin_pt=0  preci_type=Single  exp_width=8  frac_width=24  explicit_period=off  period=1  equ=P=C  opselect=C  inp2=PCIN>>17  opr=+  inp1=P  carry=CIN  dbl_ovrd=off  block_type=constant
  Constant9 : xbsIndex_r4/Constant  const=9  gui_display_data_type=Fixed-point  arith_type=Unsigned  n_bits=4  bin_pt=0  preci_type=Single  exp_width=8  frac_width=24  explicit_period=off  period=1  equ=P=C  opselect=C  inp2=PCIN>>17  opr=+  inp1=P  carry=CIN  dbl_ovrd=off  block_type=constant
  Relational{2..13} (12 alike) : xbsIndex_r4/Relational  mode=a=b  op_type=Bool  en=off  latency=0  dbl_ovrd=off  block_type=relational
  Out1 : Outport
  Out2 : Outport  Port=2
  Out3 : Outport  Port=3
  Out4 : Outport  Port=4
  Out5 : Outport  Port=5
  Out6 : Outport  Port=6
  Out7 : Outport  Port=7
  Out8 : Outport  Port=8
  Out9 : Outport  Port=9
  Out10 : Outport  Port=10
  Out11 : Outport  Port=11
  Out12 : Outport  Port=12
  wires:
  Constant1/1 -> Relational3/2
  Constant2/1 -> Relational4/2
  Relational2/1 -> Out1/1
  Relational5/1 -> Out4/1
  Relational6/1 -> Out5/1
  Relational12/1 -> Out11/1
  Relational7/1 -> Out6/1
  Relational11/1 -> Out10/1
  Relational10/1 -> Out9/1
  Relational13/1 -> Out12/1
  Constant/1 -> Relational2/2
  Constant4/1 -> Relational6/2
  Constant5/1 -> Relational7/2
  Constant6/1 -> Relational8/2
  Constant7/1 -> Relational9/2
  Constant3/1 -> Relational5/2
  Constant9/1 -> Relational11/2
  Constant8/1 -> Relational10/2
  Constant10/1 -> Relational12/2
  Constant11/1 -> Relational13/2
  Relational8/1 -> Out7/1
  Relational4/1 -> Out3/1
  Relational3/1 -> Out2/1
  Relational9/1 -> Out8/1
  In1/1 -> Relational3/1, Relational4/1, Relational6/1, Relational7/1, Relational8/1, Relational9/1, Relational10/1, Relational11/1, Relational12/1, Relational13/1, Relational5/1, Relational2/1

== system CryoDet12Chan/DspCore/AdcDac 0/SBmodulator/Phase Modulator ==
  Iin : Inport
  Qin : Inport  Port=2
  Ipm : Inport  Port=3
  Qpm : Inport  Port=4
  AddSub : xbsIndex_r4/AddSub  mode=Subtraction  use_carryin=off  use_carryout=off  en=off  latency=1  precision=User Defined  arith_type="Signed  (2's comp)"  n_bits=16  bin_pt=15  quantization=Truncate  overflow=Wrap  use_behavioral_HDL=off  hw_selection=Fabric  pipelined=off  dbl_ovrd=off  block_type=addsub
  AddSub1 : xbsIndex_r4/AddSub  mode=Addition  use_carryin=off  use_carryout=off  en=off  latency=1  precision=User Defined  arith_type="Signed  (2's comp)"  n_bits=16  bin_pt=15  quantization=Truncate  overflow=Wrap  use_behavioral_HDL=off  hw_selection=Fabric  pipelined=off  dbl_ovrd=off  block_type=addsub
  Mult{1..4} (4 alike) : xbsIndex_r4/Mult  precision=User Defined  arith_type="Signed  (2's comp)"  n_bits=16  bin_pt=15  quantization=Truncate  overflow=Wrap  en=off  latency=3  use_behavioral_HDL=off  opt=Speed  use_embedded=on  optimum_pipeline=off  pipeline=on  dbl_ovrd=off  use_rpm=on  placement_style=Triangular  block_type=mult
  Iout : Outport
  Qout : Outport  Port=2
  wires:
  Iin/1 -> Mult4/1, Mult2/1
  Qin/1 -> Mult1/1, Mult3/1
  Ipm/1 -> Mult2/2, Mult1/2
  Qpm/1 -> Mult3/2, Mult4/2
  Mult2/1 -> AddSub/1
  Mult3/1 -> AddSub/2
  Mult1/1 -> AddSub1/1
  Mult4/1 -> AddSub1/2
  AddSub/1 -> Iout/1
  AddSub1/1 -> Qout/1

== system CryoDet12Chan/DspCore/AdcDac 0/dF/CplxProd ==
  tvalidIn : Inport
  Im_A : Inport  Port=2
  Re_A : Inport  Port=3
  Im_B : Inport  Port=4
  Re_B : Inport  Port=5
  AddSub : xbsIndex_r4/AddSub  mode=Subtraction  use_carryin=off  use_carryout=off  en=off  latency=3  precision=Full  arith_type=Unsigned  n_bits=16  bin_pt=14  quantization=Truncate  overflow=Wrap  use_behavioral_HDL=off  hw_selection=DSP48  pipelined=on  dbl_ovrd=off  block_type=addsub
  AddSub1 : xbsIndex_r4/AddSub  mode=Addition  use_carryin=off  use_carryout=off  en=off  latency=3  precision=Full  arith_type=Unsigned  n_bits=16  bin_pt=14  quantization=Truncate  overflow=Wrap  use_behavioral_HDL=off  hw_selection=DSP48  pipelined=on  dbl_ovrd=off  block_type=addsub
  Delay : xbsIndex_r4/Delay  rst=off  infoeditControl=Selection of Reset will increase slice count due to use of real FFs and instead of SRLs  en=off  latency=3  reg_retiming=off  dbl_ovrd=off  block_type=delay
  Delay1 : xbsIndex_r4/Delay  rst=off  infoeditControl=Selection of Reset will increase slice count due to use of real FFs and instead of SRLs  en=off  latency=3  reg_retiming=off  dbl_ovrd=off  block_type=delay
  Mult{,1..3} (4 alike) : xbsIndex_r4/Mult  precision=Full  arith_type="Signed  (2's comp)"  n_bits=16  bin_pt=14  quantization=Truncate  overflow=Wrap  en=off  latency=3  use_behavioral_HDL=off  opt=Speed  use_embedded=on  optimum_pipeline=off  pipeline=on  dbl_ovrd=off  use_rpm=on  placement_style=Triangular  block_type=mult
  tvalidOut : Outport
  Im_Out : Outport  Port=2
  Re_Out : Outport  Port=3
  wires:
  Delay/1 -> Delay1/1
  Mult2/1 -> AddSub1/1
  Mult/1 -> AddSub/1
  Mult1/1 -> AddSub/2
  Mult3/1 -> AddSub1/2
  Re_A/1 -> Mult3/1, Mult/1
  Im_A/1 -> Mult2/1, Mult1/1
  tvalidIn/1 -> Delay/1
  Im_B/1 -> Mult1/2, Mult3/2
  Re_B/1 -> Mult/2, Mult2/2
  Delay1/1 -> tvalidOut/1
  AddSub/1 -> Re_Out/1
  AddSub1/1 -> Im_Out/1

== system CryoDet12Chan/DspCore/AdcDac 0/dF/CplxProd1 ==
  tvalidIn : Inport
  Im_A : Inport  Port=2
  Re_A : Inport  Port=3
  Im_B : Inport  Port=4
  Re_B : Inport  Port=5
  AddSub : xbsIndex_r4/AddSub  mode=Subtraction  use_carryin=off  use_carryout=off  en=off  latency=3  precision=Full  arith_type=Unsigned  n_bits=16  bin_pt=14  quantization=Truncate  overflow=Wrap  use_behavioral_HDL=off  hw_selection=DSP48  pipelined=on  dbl_ovrd=off  block_type=addsub
  AddSub1 : xbsIndex_r4/AddSub  mode=Addition  use_carryin=off  use_carryout=off  en=off  latency=3  precision=Full  arith_type=Unsigned  n_bits=16  bin_pt=14  quantization=Truncate  overflow=Wrap  use_behavioral_HDL=off  hw_selection=DSP48  pipelined=on  dbl_ovrd=off  block_type=addsub
  Delay : xbsIndex_r4/Delay  rst=off  infoeditControl=Selection of Reset will increase slice count due to use of real FFs and instead of SRLs  en=off  latency=3  reg_retiming=off  dbl_ovrd=off  block_type=delay
  Delay1 : xbsIndex_r4/Delay  rst=off  infoeditControl=Selection of Reset will increase slice count due to use of real FFs and instead of SRLs  en=off  latency=3  reg_retiming=off  dbl_ovrd=off  block_type=delay
  Mult{,1..3} (4 alike) : xbsIndex_r4/Mult  precision=Full  arith_type="Signed  (2's comp)"  n_bits=16  bin_pt=14  quantization=Truncate  overflow=Wrap  en=off  latency=3  use_behavioral_HDL=off  opt=Speed  use_embedded=on  optimum_pipeline=off  pipeline=on  dbl_ovrd=off  use_rpm=on  placement_style=Triangular  block_type=mult
  tvalidOut : Outport
  Im_Out : Outport  Port=2
  Re_Out : Outport  Port=3
  wires:
  Delay/1 -> Delay1/1
  Mult2/1 -> AddSub1/1
  Mult/1 -> AddSub/1
  Mult1/1 -> AddSub/2
  Mult3/1 -> AddSub1/2
  Re_A/1 -> Mult3/1, Mult/1
  Im_A/1 -> Mult2/1, Mult1/1
  tvalidIn/1 -> Delay/1
  Im_B/1 -> Mult1/2, Mult3/2
  Re_B/1 -> Mult/2, Mult2/2
  Delay1/1 -> tvalidOut/1
  AddSub/1 -> Re_Out/1
  AddSub1/1 -> Im_Out/1

== system CryoDet12Chan/DspCore/AdcDac 0/dF/etaRAM ==
  note: 4 May 2016 Now floating point
  readAddr : Inport
  "etaBusIn " : Inport  Port=2
  Bus Selector : BusSelector  OutputSignals=channel,etaQ,etaI
  Concat : xbsIndex_r4/Concat  num_inputs=2  dbl_ovrd=off  block_type=concat
  Dual Port RAM : xbsIndex_r4/Dual Port RAM  depth=2^freqBusAddrBits  initVector=0  distributed_mem=Block RAM  init_a=0  init_b=0  rst_a=off  rst_b=off  en_a=off  en_b=off  latency=2  write_mode_A=Read Before Write  write_mode_B=Read After Write  optimize=Area  dbl_ovrd=off  block_type=dpram
  Gateway Out{1..3,13,26,29} (6 alike) : xbsIndex_r4/Gateway Out  inherit_from_input=off  hdl_port=off  rows=1  columns=1  UseAsDAC=off  DACChannel='1'  interface=None  automatic_assignment=on  address_offset=hex2dec('00')  intf_name=''  intf_description=''  timing_constraint=None  locs_specified=off  LOCs={}  io_standard={}  block_type=gatewayout
  Mux1 : Mux  Inputs=2
  Mux13 : Mux  Inputs=2
  Mux7 : Mux  Inputs=2
  Reinterpret : xbsIndex_r4/Reinterpret  force_arith_type=on  arith_type=Unsigned  force_bin_pt=on  bin_pt=0  block_type=reinterpret
  Reinterpret1 : xbsIndex_r4/Reinterpret  force_arith_type=on  arith_type=Unsigned  force_bin_pt=on  bin_pt=0  block_type=reinterpret
  Reinterpret2 : xbsIndex_r4/Reinterpret  force_arith_type=on  arith_type=Floating-point  force_bin_pt=on  bin_pt=24  block_type=reinterpret
  Reinterpret3 : xbsIndex_r4/Reinterpret  force_arith_type=on  arith_type=Floating-point  force_bin_pt=on  bin_pt=24  block_type=reinterpret
  Slice : xbsIndex_r4/Slice  nbits=32  boolean_output=off  mode=Upper Bit Location + Width  bit1=0  base1=MSB of Input  bit0=0  base0=LSB of Input  dbl_ovrd=off  block_type=slice
  Slice1 : xbsIndex_r4/Slice  nbits=32  boolean_output=off  mode=Lower Bit Location + Width  bit1=0  base1=MSB of Input  bit0=0  base0=LSB of Input  dbl_ovrd=off  block_type=slice
  Terminator3 : Terminator
  eta ram in out : Scope  NumInputPorts=3
  read : xbsIndex_r4/Constant  const=0  gui_display_data_type=Boolean  arith_type=Boolean  n_bits=16  bin_pt=14  preci_type=Single  exp_width=8  frac_width=24  explicit_period=off  period=1  equ=P=C  opselect=C  inp2=PCIN>>17  opr=+  inp1=P  carry=CIN  dbl_ovrd=off  block_type=constant
  write : xbsIndex_r4/Constant  const=1.0  gui_display_data_type=Boolean  arith_type=Boolean  n_bits=16  bin_pt=14  preci_type=Single  exp_width=8  frac_width=24  explicit_period=off  period=1  equ=P=C  opselect=C  inp2=PCIN>>17  opr=+  inp1=P  carry=CIN  dbl_ovrd=off  block_type=constant
  etaQ : Outport
  etaI : Outport  Port=2
  wires:
  read/1 -> Dual Port RAM/6
  Bus Selector/1 -> Gateway Out26/1, Dual Port RAM/1  "<channel>"
  write/1 -> Dual Port RAM/3
  Dual Port RAM/2 -> Slice1/1, Slice/1
  Dual Port RAM/1 -> Terminator3/1
  "etaBusIn "/1 -> Bus Selector/1
  Bus Selector/2 -> Gateway Out2/1, Reinterpret/1  "<etaQ>"
  Bus Selector/3 -> Gateway Out29/1, Reinterpret1/1  "<etaI>"
  Reinterpret1/1 -> Concat/2
  Reinterpret/1 -> Concat/1
  Concat/1 -> Dual Port RAM/2, Dual Port RAM/5
  Slice/1 -> Reinterpret2/1
  Slice1/1 -> Reinterpret3/1
  Reinterpret2/1 -> Gateway Out1/1, etaQ/1
  Reinterpret3/1 -> Gateway Out3/1, etaI/1
  Gateway Out29/1 -> Mux13/1
  Mux13/1 -> eta ram in out/2
  Gateway Out13/1 -> Mux7/2
  Gateway Out26/1 -> Mux7/1
  Mux7/1 -> eta ram in out/1
  Gateway Out2/1 -> Mux13/2
  readAddr/1 -> Gateway Out13/1, Dual Port RAM/4
  Gateway Out3/1 -> Mux1/1
  Mux1/1 -> eta ram in out/3
  Gateway Out1/1 -> Mux1/2
